simulink model "scara_robot_foward"  (R2023a)
settings: Solver=FixedStepAuto  StartTime=0.0  StopTime=5  FixedStep=0.001  RelTol=1e-3
InitFcn:
  | % Create the Simulink.Parameter objects
  | length1_param = Simulink.Parameter;
  | length2_param = Simulink.Parameter;
  | 
  | % Set the values
  | length1_param.Value = 1.56;  % replace with your value
  | length2_param.Value = 2.56;  % replace with your value
  | 
  | % Set the properties to make them tunable
  | length1_param.CoderInfo.StorageClass = 'ExportedGlobal';
  | length2_param.CoderInfo.StorageClass = 'ExportedGlobal';
  | 
  | % Set the data type
  | length1_param.DataType = 'double';
  | length2_param.DataType = 'double';
model workspace (MAT data in the model file):
  rigidBodyTree = 0
libraries: robotmaniplib x1
settings Model: Creator=divij  LastModifiedBy=divij
settings DataIOCC: SaveFormat=Structure
settings OptimizationCC: DefaultParameterBehavior=Inlined  UseDivisionForNetSlopeComputation=on  GainParamInheritBuiltInType=on  UseFloatMulNetSlope=on  OptimizeBlockIOStorage=off  ZeroExternalMemoryAtStartup=off  ZeroInternalMemoryAtStartup=off  LifeSpan=1  OptimizeDataStoreBuffers=off  BusAssignmentInplaceUpdate=off
settings DebuggingCC: SFUnexpectedBacktrackingDiag=warning  SFNoUnconditionalDefaultTransitionDiag=warning
settings HardwareCC: ProdLongLongMode=on
settings RTWCC: PackageGeneratedCodeAndArtifacts=on  GenerateReport=on  Toolchain=Catkin  BuildConfiguration=Debug  LaunchReport=on  TargetLang=C++
settings CodeAppCC: ForceParamTrailComments=on  MATLABSourceComments=on  EnableCustomComments=on
settings GRTTargetCC: TargetLangStandard=C++11 (ISO)  CombineSignalStateStructs=on  CodeInterfacePackaging=C++ class  SupportVariableSizeSignals=on  MultiInstanceErrorCode=Warning

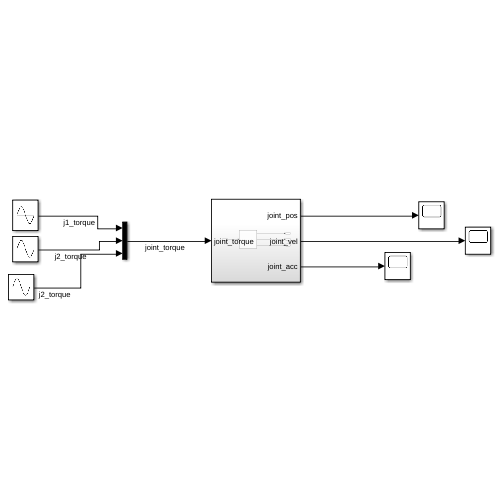
[thumbnail: Simulink's stored preview of the top-level diagram]
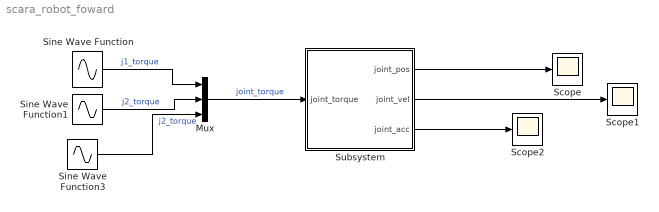
== system scara_robot_foward ==
  Mux : Mux  Inputs=3
  Scope : Scope
  Scope1 : Scope
  Scope2 : Scope
  Sine Wave Function : Sin  Amplitude=0  SampleTime=0
  Sine Wave Function1 : Sin  Amplitude=0  SampleTime=0
  Sine Wave Function3 : Sin  Amplitude=0.5  SampleTime=0
  Subsystem : Subsystem
  wires:
  Sine Wave Function1/1 -> Mux/2  "j2_torque"
  Sine Wave Function/1 -> Mux/1  "j1_torque"
  Mux/1 -> Subsystem/1(joint_torque)  "joint_torque"
  Subsystem/1(joint_pos) -> Scope/1
  Subsystem/2(joint_vel) -> Scope1/1
  Subsystem/3(joint_acc) -> Scope2/1
  Sine Wave Function3/1 -> Mux/3  "j2_torque"

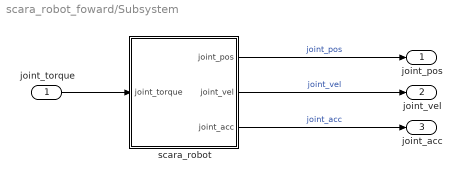
== system scara_robot_foward/Subsystem ==
  joint_torque : Inport
  scara_robot : Subsystem  TreatAsAtomicUnit=on
  joint_pos : Outport
  joint_vel : Outport  Port=2
  joint_acc : Outport  Port=3
  wires:
  scara_robot/3(joint_acc) -> joint_acc/1  "joint_acc"
  scara_robot/2(joint_vel) -> joint_vel/1  "joint_vel"
  scara_robot/1(joint_pos) -> joint_pos/1  "joint_pos"
  joint_torque/1 -> scara_robot/1(joint_torque)

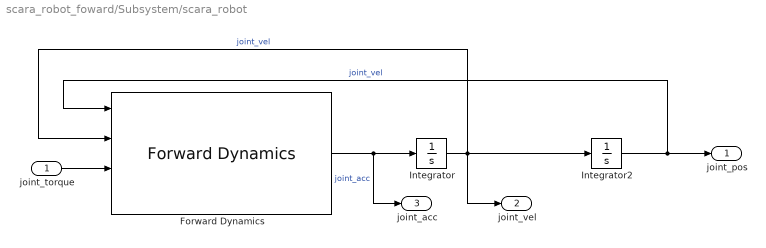
== system scara_robot_foward/Subsystem/scara_robot ==
  joint_torque : Inport
  Forward Dynamics : robotmaniplib/Forward Dynamics  RigidBodyTree=robot  SimulateUsing=Interpreted execution
  Integrator : Integrator  UpperSaturationLimit=10  LowerSaturationLimit=-10
  Integrator2 : Integrator  LimitOutput=on  UpperSaturationLimit=pi/2  LowerSaturationLimit=-pi/2
  joint_pos : Outport
  joint_vel : Outport  Port=2
  joint_acc : Outport  Port=3
  wires:
  Forward Dynamics/1 -> joint_acc/1, Integrator/1  "joint_acc"
  Integrator/1 -> Integrator2/1, joint_vel/1, Forward Dynamics/2  "joint_vel"
  joint_torque/1 -> Forward Dynamics/3
  Integrator2/1 -> Forward Dynamics/1, joint_pos/1  "joint_vel"
